simulink model "Complete_Assembly_ACC"  (R2024a)
settings: Solver=VariableStepAuto  StartTime=0.0  StopTime=30  RelTol=1e-3
libraries: autolibshared x2, sim3dautolib x2, dspstat3 x2, dspsigops x2, sim3dprobsensorlib x2, mpcadaslib x1, trackingutilitieslib x1, drivinglib x1, sim3dcameralib x1, sim3dphyssensorlib x1, sim3dlib x1, drivingsim3d x1
settings Model: Creator=moata  LastModifiedBy=moata

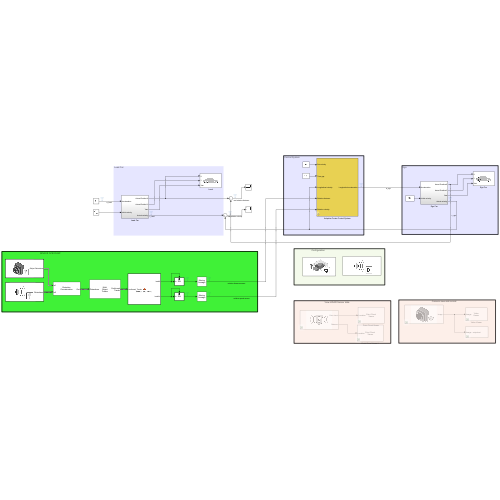
[thumbnail: Simulink's stored preview of the top-level diagram]
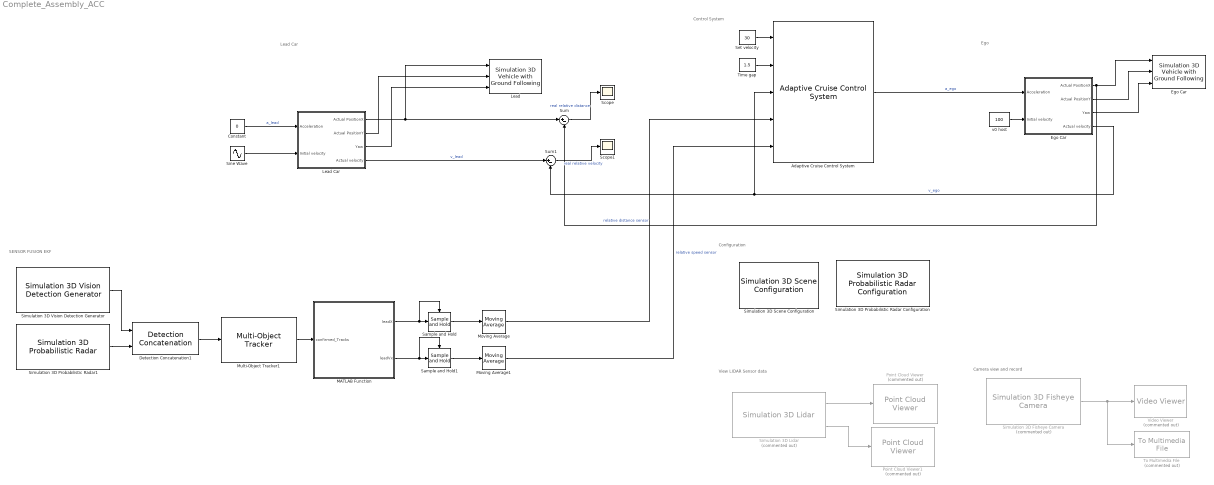
== system Complete_Assembly_ACC ==
  note: Camera view and record
  note: Control System
  note: View LIDAR Sensor data
  note: Ego
  note: Lead Car
  note: SENSOR FUSION EKF
  note: Configuration
  Adaptive Cruise Control System : mpcadaslib/Adaptive Cruise Control System  EgoModel=tf(1,[0.5,1,0])  InitialEgoVelocity=20  DefaultSpacing=40  MaxVelocity=50  MinAcceleration=-5  amin_ext=off  MaxAcceleration=5  amax_ext=off  Ts=0.1  PredictionHorizon=50  ControllerBehavior=0.500  suboptimal=off  maxiter=10  datatypeopt=double  optmode=off  trackmode=off
  Constant : Constant  Value=0
  Detection Concatenation1 : trackingutilitieslib/Detection Concatenation  NumInputs=2  BusNameSource=Auto  BusName=BusDetectionConcatenation  SimulateUsing=Interpreted execution
      settings: LibrarySourceBlock=drivinglib/Detection Concatenation
  Ego Car : Subsystem
  "Ego Car " : sim3dautolib/Simulation 3D Vehicle with Ground Following  Priority=-1  PassVehMesh=Muscle car  MeshPath=/MathWorksAutomotiveContent/Vehicles/Muscle/Meshes/SK_MuscleCar.SK_MuscleCar  TrackWidth=1.9  WheelBase=3  WheelRadius=0.35  VehColor=Black  InitialPos=[80, 0, 0]  InitialRot=[0, 0, 0]  ActorName=SimulinkVehicle1  SampleTime=-1  ActorType=SimulinkVehicle  ID=1  aMode=3  ActorTag=SimulinkVehicle1  CoordinateScheme=ISO  VehLightsControl=off  HeadlightColor=[ 1, 1, 1 ]  HighBeamIntensity=100000  LowBeamIntensity=60000  HighBeamConeAngle=70  LowBeamConeAngle=70  LeftHeadlightOrientation=[ 0, 0 ]  RightHeadlightOrientation=[ 0, 0 ]  BrakelightIntensity=500  ReverselightIntensity=500  SignallightIntensity=500  SignallightPeriod=1  SignalPulseWidth=50  TransformOutportEnabled=off
      settings: LibrarySourceBlock=drivingsim3d/Simulation 3D Vehicle with Ground Following
  Lead : sim3dautolib/Simulation 3D Vehicle with Ground Following  Priority=-1  PassVehMesh=Box truck  MeshPath=/MathWorksAutomotiveContent/Vehicles/Muscle/Meshes/SK_MuscleCar.SK_MuscleCar  TrackWidth=1.9  WheelBase=3  WheelRadius=0.35  VehColor=Silver  InitialPos=[80, 0, 0]  InitialRot=[0, 0, 0]  ActorName=SimulinkVehicle2  SampleTime=-1  ActorType=SimulinkVehicle  ID=2  aMode=3  ActorTag=SimulinkVehicle2  CoordinateScheme=ISO  VehLightsControl=off  HeadlightColor=[ 1, 1, 1 ]  HighBeamIntensity=100000  LowBeamIntensity=60000  HighBeamConeAngle=70  LowBeamConeAngle=70  LeftHeadlightOrientation=[ 0, 0 ]  RightHeadlightOrientation=[ 0, 0 ]  BrakelightIntensity=500  ReverselightIntensity=500  SignallightIntensity=500  SignallightPeriod=1  SignalPulseWidth=50  TransformOutportEnabled=off
      settings: LibrarySourceBlock=drivingsim3d/Simulation 3D Vehicle with Ground Following
  Lead Car : Subsystem
  MATLAB Function : MATLAB Function  TreatAsAtomicUnit=on
  Moving Average : dspstat3/Moving Average  Method=Sliding window  ForgettingFactorPort=off  SpecifyWindowLength=on  WindowLength=20  OverlapLength=19  AllowArbitraryInputLength=off  ForgettingFactor=0.8  SimulateUsing=Interpreted execution
  Moving Average1 : dspstat3/Moving Average  Method=Sliding window  ForgettingFactorPort=off  SpecifyWindowLength=on  WindowLength=20  OverlapLength=19  AllowArbitraryInputLength=off  ForgettingFactor=0.8  SimulateUsing=Interpreted execution
  Multi-Object Tracker1 : drivinglib/Multi-Object Tracker  TrackerIndex=uint32( 0 )  FilterInitializationFcn=initcvekf  AssignmentThreshold=30  ConfirmationThreshold=[ 2, 3 ]  DeletionThreshold=[ 5, 5 ]  MaxNumTracks=20  MaxNumSensors=2  OOSMHandling=Neglect  StateParametersSimulink=struct  HasStateParametersInput=off  TimeInputSource=Auto  HasCostMatrixInput=off  HasDetectableTrackIDsInput=off  BusNameSource=Property  BusName=BusMultiObjectTracker1  TentativeTracksOutputPort=off  AllTracksOutputPort=off  SimulateUsing=Interpreted execution
  Point Cloud Viewer : PointCloudViewer  Commented=on  FigPos=[989.8 733.2 409.6 300]
  Point Cloud Viewer1 : PointCloudViewer  Commented=on  FigPos=[989.8 733.2 409.6 300]
  Sample and Hold : dspsigops/Sample and Hold  trig=Rising edge  initCond=0  latchinput=off
  Sample and Hold1 : dspsigops/Sample and Hold  trig=Rising edge  initCond=0  latchinput=off
  Scope : Scope
  Scope1 : Scope
  Set velocity : Constant  Value=30  SampleTime=0.1
  Simulation 3D Fisheye Camera : sim3dcameralib/Simulation 3D Fisheye Camera  Priority=1  Commented=on  sensorTag=Sim3dSensor1  sensorId=1  sensorName=Sim3dSensor1  vehTagList={'Scene Origin';'SimulinkVehicle1';'SimulinkVehicle2'}  vehTag=SimulinkVehicle1  mountLoc=Front bumper  offsetFlag=off  tmountOffset=[0, 0, 0]  extTmount=off  rmountOffset=[0, 0, 0]  extRmount=off  OpticalCenter=[640, 360]  ImageSize=[720, 1280]  RadialDistortion=[320, 0, 0, 0]  StretchMatrix=[1, 0; 0, 1]  TransformOutportEnabled=off  SampleTime=-1  mountPoint=[2.47350001335144 0 0.439999997615814]  mountOrientation=[0 0 0]  aMode=3  ID=1
      settings: LibrarySourceBlock=drivingsim3d/Simulation 3D Fisheye Camera
  Simulation 3D Lidar : sim3dphyssensorlib/Simulation 3D Lidar  Priority=1  Commented=on  sensorTag=Sim3dSensor2  sensorId=2  sensorName=Sim3dSensor2  vehTagList={'Scene Origin';'SimulinkVehicle1';'SimulinkVehicle2'}  vehTag=SimulinkVehicle1  mountLoc=Hood center  offsetFlag=off  tmountOffset=[0, 0, 0]  rmountOffset=[0, 0, 0]  DetectionRange=120  RangeResolution=0.002  VerticalFOV=40  VerticalResolution=1.25  HorizontalFOV=360  HorizontalResolution=0.16  DistanceOutportEnabled=on  ReflectivityOutportEnabled=off  SemanticOutportEnabled=off  TransformOutportEnabled=off  SampleTime=-1  mountPoint=[1.27600002288818 0 1.12999999523163]  mountOrientation=[0 0 0]  aMode=3  ID=2
      settings: LibrarySourceBlock=drivingsim3d/Simulation 3D Lidar
  Simulation 3D Probabilistic Radar Configuration : sim3dprobsensorlib/Simulation 3D Probabilistic Radar Configuration  RCSactorKeys=[10]  RCSactorProfiles={[20, 25 ; 15, 30]}  RCSdefaultValue=-20  aMode=3
      settings: LibrarySourceBlock=drivingsim3d/Simulation 3D Probabilistic Radar Configuration
  Simulation 3D Probabilistic Radar1 : sim3dprobsensorlib/Simulation 3D Probabilistic Radar  Priority=1  sensorTag=Sim3dSensor3  sensorId=3  sensorName=Sim3dSensor3  vehTagList={'Scene Origin';'SimulinkVehicle1';'SimulinkVehicle2'}  vehTag=SimulinkVehicle1  mountLoc=Front bumper  offsetFlag=off  tmountOffset=[0, 0, 0]  rmountOffset=[0, 0, 0]  AzimuthResolution=4  ElevationResolution=5  RangeResolution=2.5  RangeRateResolution=0.5  AzimuthBiasFraction=0.1  ElevationBiasFraction=0.1  RangeBiasFraction=0.05  RangeRateBiasFraction=0.05  FieldOfView=[ 20, 5 ]  DetectionRange=[ 1, 500 ]  RangeRateLimits=[ -100, 100 ]  DetectionProbability=0.95  FalseAlarmRate=1e-7  ReferenceRange=500  ReferenceRCS=20  HasElevation=on  HasRangeRate=on  HasNoise=off  HasFalseAlarms=off  InitialSeedSource=Repeatable  InitialSeed=0  MaxNumDetections=150  DetectionCoordinates=Ego Cartesian  SpecifyOutputBusName=off  BusName=BusSimulation3DRadarTruthSensor  SampleTime=-1  mountPoint=[2.47350001335144 0 0.439999997615814]  mountOrientation=[0 0 0]  aMode=3  ID=3
      settings: LibrarySourceBlock=drivingsim3d/Simulation 3D Probabilistic Radar
  Simulation 3D Scene Configuration : sim3dlib/Simulation 3D Scene Configuration  Priority=0  ProjectFormat=Default Scenes  SceneDesc=Straight road  ProjectName=C:\Program Files\MATLAB\R2024a\toolbox\shared\sim3d_projects\automotive_project_windows\UE\WindowsNoEditor\VehicleSimulation.exe  ScenePath=/Game/Maps/HwStrght  EnableOpenDRIVE=off  vehTagList={'Scene Origin';'SimulinkVehicle1';'SimulinkVehicle2'}  vehTag=SimulinkVehicle1  FreeCameraInitialTranslation=[0, 0, 0]  FreeCameraDefaultInitialTranslation=[-6, 0, 2]  FreeCameraInitialRotation=[0, 0, 0]  FreeCameraDefaultInitialRotation=[0, -15, 0]  OpVisEn=off  Ts=1/60  EnableWindow=on  EnableRemoteAccess=off  EnableWeather=off  SunAzimuth=90  SunAltitude=40.0  EnableGeospatialSun=off  Latitude=0  Longitude=0  Date=2023-01-01  Time=10:30:00  GeoTimeZone=-5.0  SunDaylightSaving=off  wind=1  clouds=10  EnableVolumetricClouds=off  CloudCoverage=0  CloudAltitude=6  fog=0  rain=0  RaindropsEffect=off  SnowDensity=0  EnableGeospatial=off  UseTrueOrigin=off  OriginHeight=200  OriginLatitude=40.744652  OriginLongitude=-73.988864  MapStyle=Aerial  AdditionalAssetIDs=[]  UseAdvancedSunSky=off  SolarTime=11  TimeZone=-5  Day=21  Month=9  Year=2022  UseDaylightSavingTime=on  DSTStartDay=10  DSTStartMonth=3  DSTEndDay=3  DSTEndMonth=11  DSTSwitchHour=2  sensorTag=MainCamera1  sensorId=1  sensorName=MainCamera1  mountLoc=Origin  offsetFlag=off  tmountOffset=[0, 0, 0]  rmountOffset=[0, 0, 0]  HorizontalResolution=1280  VerticalResolution=720  HorizontalFOV=60  mountPoint=[0 0 0]  mountOrientation=[0 0 0]  aMode=3  ID=1  GeoTrigger=Inactive
      settings: LibrarySourceBlock=drivingsim3d/Simulation 3D Scene Configuration
  Simulation 3D Vision Detection Generator : drivingsim3d/Simulation 3D Vision Detection Generator  Priority=1  sensorTag=Sim3dSensor255  sensorId=4  sensorName=Sim3dSensor2  vehTagList={'Scene Origin';'SimulinkVehicle1';'SimulinkVehicle2'}  vehTag=SimulinkVehicle1  mountLoc=Front bumper  offsetFlag=off  tmountOffset=[0, 0, 0]  rmountOffset=[0, 0, 0]  DetectorOutput=Objects only  MaxNumDetections=50  MaxNumLanes=30  laneSampleDistances=0:0.5:9.5  BusNameSource=Auto  BusName=BusObjectDetections  BusName2Source=Auto  BusName2=BusLaneDetections  MaxRange=500  BoundingBoxAccuracy=5  ProcessNoiseIntensity=5  MaxSpeed=50  MaxAllowedOcclusion=0.5  MinObjectImageSize=[ 15, 15 ]  DetectionProbability=0.9  FalsePositivesPerImage=0  MinLaneImageSize=[ 20, 3 ]  LaneBoundaryAccuracy=3  HasNoise=off  InitialSeedSource=Repeatable  InitialSeed=1  uniqueActorIdentifier=[]  actorClassInteger=0  cuboidLength=4.7  cuboidWidth=1.8  cuboidHeight=1.4  rotationalCenter={[-1.35, 0, 0]}  focalLength=[800, 800]  opticalCenter=[320, 240]  imageSize=[480, 640]  radialDistortionCoefficients=[0, 0]  tangentialDistortionCoefficients=[0, 0]  cameraAxisSkew=0  actorTruthOutportEnabled=off  laneTruthOutportEnabled=off  SampleTime=-1  checkedSampleTime=0.016667  mountPoint=[2.47350001335144 0 0.439999997615814]  mountOrientation=[0 0 0]  aMode=3  ID=4
  Sine Wave : Sin  Amplitude=20  Bias=50  Frequency=0.5  SampleTime=0
  Sum : Sum  Inputs=|+-
  Sum1 : Sum  Inputs=|+-
  Time gap : Constant  Value=1.5  SampleTime=0.1
  To Multimedia File : dspvision/To Multimedia File  Commented=on  outputFilename=C:\Users\moata\Desktop\output.avi  streamSelection=Video only  videoCompressor=None (uncompressed)  audioCompressor=None (uncompressed)  imagePorts=One multidimensional signal  fileType=AVI  audioDatatype=Determine from input data type  fourcc=RGB  audioBitRate=128  audioQuality=75  videoQuality=75  mj2000CompFactor=10
      settings: LibrarySourceBlock=visionsinks/To Multimedia File
  Video Viewer : VideoViewer  Commented=on  FigPos=[931.4 762.8 482.4 364.8]
  v0 host : Constant  Value=100  SampleTime=0.1
  wires:
  Time gap/1 -> Adaptive Cruise Control System/2
  Lead Car/1(Actual PositionX) -> Sum/1, Lead/1
  Lead Car/4(Actual velocity) -> Sum1/1  "v_lead"
  Simulation 3D Lidar/2 -> Point Cloud Viewer1/1
  v0 host/1 -> Ego Car/2(Initial velocity)
  Ego Car/1(Actual PositionX) -> "Ego Car "/1, Sum/2
  Simulation 3D Lidar/1 -> Point Cloud Viewer/1
  Simulation 3D Fisheye Camera/1 -> Video Viewer/1, To Multimedia File/1
  Set velocity/1 -> Adaptive Cruise Control System/1
  Lead Car/3(Yaw) -> Lead/3
  Adaptive Cruise Control System/1 -> Ego Car/1(Acceleration)  "a_ego"
  Ego Car/2(Actual PositionY) -> "Ego Car "/2
  Constant/1 -> Lead Car/1(Acceleration)  "a_lead"
  Ego Car/4(Actual velocity) -> Adaptive Cruise Control System/3, Sum1/2  "v_ego"
  Lead Car/2(Actual PositionY) -> Lead/2
  Ego Car/3(Yaw) -> "Ego Car "/3
  Sine Wave/1 -> Lead Car/2(Initial velocity)
  Simulation 3D Vision Detection Generator/1 -> Detection Concatenation1/1
  Detection Concatenation1/1 -> Multi-Object Tracker1/1
  Simulation 3D Probabilistic Radar1/1 -> Detection Concatenation1/2
  MATLAB Function/1(leadX) -> Sample and Hold/Trigger, Sample and Hold/1
  Multi-Object Tracker1/1 -> MATLAB Function/1(confirmed_Tracks)
  Sample and Hold/1 -> Moving Average/1
  Sample and Hold1/1 -> Moving Average1/1
  MATLAB Function/2(leadVx) -> Sample and Hold1/Trigger, Sample and Hold1/1
  Moving Average/1 -> Adaptive Cruise Control System/4  "relative distance sensor"
  Moving Average1/1 -> Adaptive Cruise Control System/5  "relative speed sensor"
  Sum/1 -> Scope/1  "real relative distance"
  Sum1/1 -> Scope1/1  "real relative velocity"

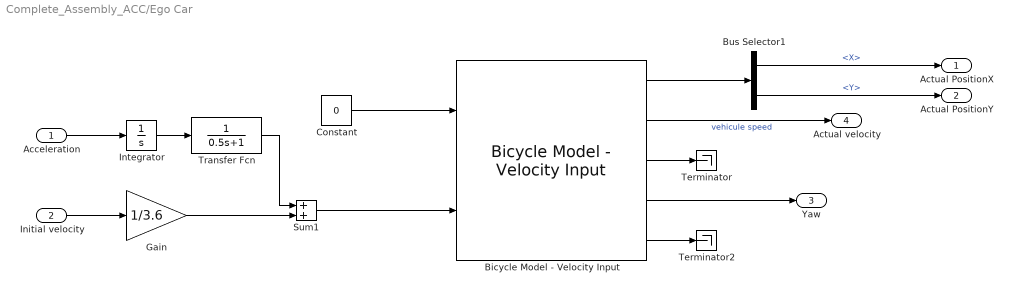
== system Complete_Assembly_ACC/Ego Car ==
  Acceleration : Inport
  Initial velocity : Inport  Port=2
  Bicycle Model - Velocity Input : autolibshared/Bicycle Model - Velocity Input  trackMode=Single (bicycle)  inputMode=External longitudinal velocity  frontSteerMode=on  rearSteerMode=off  windMode=off  muMode=off  extFMode=off  extMMode=off  aMode=3  NF=2  NR=2  m=2000  a=1.4  b=1.6  h=0.35  X_o=0  xdot_o=0  CalphaMode=off  sigmaMode=on  w=[1.4,1.4]  Cy_f=12e3  Cy_r=11e3  sigma_f=.1  sigma_r=.1  alpha_f_brk=[-.1 .1]  Cy_f_data=[-9e3 9e3]  alpha_r_brk=[-.1 .1]  Cy_r_data=[-9e3 9e3]  Y_o=0  ydot_o=0  Izz=4000  psi_o=0  r_o=0  Af=2  Cd=.3  Cl=.1  Cpm=.1  beta_w=[0 0.01:0.01:0.3]  Cs=[0 0.01:0.01:0.3]  Cym=[0 1e-6:0.01:0.3]  Pabs=101325  Tair=273  g=9.81  mu=1  xdot_tol=.01  Fznom=5000  Fxtire_sat=1e6  Fytire_sat=1e6  longOff=0  latOff=0  vertOff=0
      settings: LibrarySourceBlock=drivingscenarioandsensors/Bicycle Model - Velocity Input
  Bus Selector1 : BusSelector  OutputSignals=InertFrm.Cg.Disp.X,InertFrm.Cg.Disp.Y
  Constant : Constant  Value=0
  Gain : Gain  Gain=1/3.6
  Integrator : Integrator
  Sum1 : Sum
  Terminator : Terminator
  Terminator2 : Terminator
  Transfer Fcn : TransferFcn  Denominator=[0.5 1]
  Actual PositionX : Outport  VectorParamsAs1DForOutWhenUnconnected=off
  Actual PositionY : Outport  Port=2  VectorParamsAs1DForOutWhenUnconnected=off
  Yaw : Outport  Port=3  VectorParamsAs1DForOutWhenUnconnected=off
  Actual velocity : Outport  Port=4  VectorParamsAs1DForOutWhenUnconnected=off
  wires:
  Initial velocity/1 -> Gain/1
  Bicycle Model - Velocity Input/3 -> Terminator/1
  Bicycle Model - Velocity Input/4 -> Yaw/1
  Bicycle Model - Velocity Input/5 -> Terminator2/1
  Bicycle Model - Velocity Input/2 -> Actual velocity/1  "vehicule speed"
  Bicycle Model - Velocity Input/1 -> Bus Selector1/1
  Constant/1 -> Bicycle Model - Velocity Input/1
  Acceleration/1 -> Integrator/1
  Sum1/1 -> Bicycle Model - Velocity Input/2
  Integrator/1 -> Transfer Fcn/1
  Transfer Fcn/1 -> Sum1/1
  Bus Selector1/1 -> Actual PositionX/1  "<X>"
  Bus Selector1/2 -> Actual PositionY/1  "<Y>"
  Gain/1 -> Sum1/2

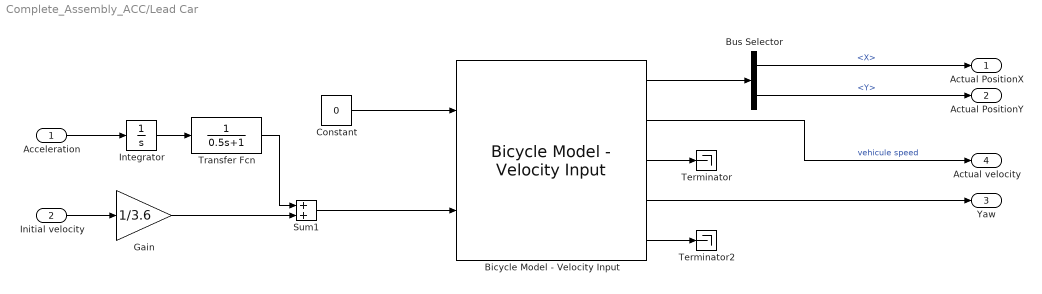
== system Complete_Assembly_ACC/Lead Car ==
  Acceleration : Inport
  Initial velocity : Inport  Port=2
  Bicycle Model - Velocity Input : autolibshared/Bicycle Model - Velocity Input  trackMode=Single (bicycle)  inputMode=External longitudinal velocity  frontSteerMode=on  rearSteerMode=off  windMode=off  muMode=off  extFMode=off  extMMode=off  aMode=3  NF=2  NR=2  m=2000  a=1.4  b=1.6  h=0.35  X_o=80  xdot_o=0  CalphaMode=off  sigmaMode=on  w=[1.4,1.4]  Cy_f=12e3  Cy_r=11e3  sigma_f=.1  sigma_r=.1  alpha_f_brk=[-.1 .1]  Cy_f_data=[-9e3 9e3]  alpha_r_brk=[-.1 .1]  Cy_r_data=[-9e3 9e3]  Y_o=0  ydot_o=0  Izz=4000  psi_o=0  r_o=0  Af=2  Cd=.3  Cl=.1  Cpm=.1  beta_w=[0 0.01:0.01:0.3]  Cs=[0 0.01:0.01:0.3]  Cym=[0 1e-6:0.01:0.3]  Pabs=101325  Tair=273  g=9.81  mu=1  xdot_tol=.01  Fznom=5000  Fxtire_sat=1e6  Fytire_sat=1e6  longOff=0  latOff=0  vertOff=0
      settings: LibrarySourceBlock=drivingscenarioandsensors/Bicycle Model - Velocity Input
  Bus Selector : BusSelector  OutputSignals=InertFrm.Cg.Disp.X,InertFrm.Cg.Disp.Y
  Constant : Constant  Value=0
  Gain : Gain  Gain=1/3.6
  Integrator : Integrator
  Sum1 : Sum
  Terminator : Terminator
  Terminator2 : Terminator
  Transfer Fcn : TransferFcn  Denominator=[0.5 1]
  Actual PositionX : Outport  VectorParamsAs1DForOutWhenUnconnected=off
  Actual PositionY : Outport  Port=2  VectorParamsAs1DForOutWhenUnconnected=off
  Yaw : Outport  Port=3  VectorParamsAs1DForOutWhenUnconnected=off
  Actual velocity : Outport  Port=4  VectorParamsAs1DForOutWhenUnconnected=off
  wires:
  Transfer Fcn/1 -> Sum1/1
  Integrator/1 -> Transfer Fcn/1
  Sum1/1 -> Bicycle Model - Velocity Input/2
  Acceleration/1 -> Integrator/1
  Constant/1 -> Bicycle Model - Velocity Input/1
  Bicycle Model - Velocity Input/1 -> Bus Selector/1
  Bus Selector/1 -> Actual PositionX/1  "<X>"
  Bicycle Model - Velocity Input/2 -> Actual velocity/1  "vehicule speed"
  Bicycle Model - Velocity Input/5 -> Terminator2/1
  Bicycle Model - Velocity Input/4 -> Yaw/1
  Bicycle Model - Velocity Input/3 -> Terminator/1
  Initial velocity/1 -> Gain/1
  Bus Selector/2 -> Actual PositionY/1  "<Y>"
  Gain/1 -> Sum1/2

== matlab function Complete_Assembly_ACC/MATLAB Function ==
  data: confirmed_Tracks input; leadX output; leadVx output
function [leadX, leadVx] = extractLeadCarInfo(confirmed_Tracks)
    
    leadX = confirmed_Tracks.Tracks(1).State(1);
    leadVx = confirmed_Tracks.Tracks(1).State(2); % X velocity

end
